simulink model "adaptive_backstepping_compliant_two_motor"  (R2022b)
settings: Solver=VariableStepAuto  StartTime=0.0  StopTime=80  RelTol=1e-3
values from neighbouring files (symbols this model uses):
  Lamda = 0.1*eye(2)    [init.m]
undefined symbols (not defined in the file or in its folder): D, J
settings Model: Creator=alexi  LastModifiedBy=alexi

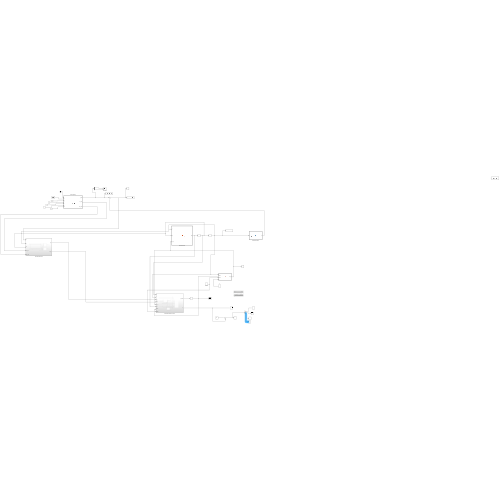
[thumbnail: Simulink's stored preview of the top-level diagram]
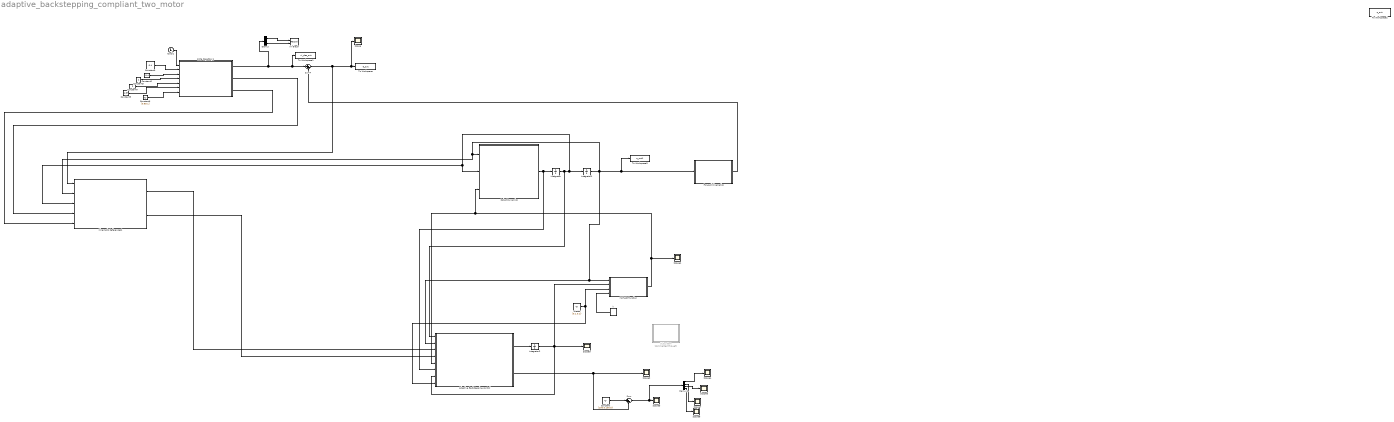
== system adaptive_backstepping_compliant_two_motor ==
  Adaptive Backstepping control : Subsystem
  Clock1 : Clock
  Constant : Constant  Value=[100,0,100,0]'
  Constant2 : Constant  Value=0.4
  Constant3 : Constant
  Constant4 : Constant  Value=2
  Constant5 : Constant  Value=1.57
  Constant6 : Constant  Value=[0.85,1]
  Constant9 : Constant  Value=0.4
  Demux : Demux  Outputs=2
  Demux1 : Demux
  Forward Kinematics : MATLAB Function  TreatAsAtomicUnit=on
  Integrator : Integrator  InitialCondition=[0,0]'
  Integrator1 : Integrator  InitialCondition=[0.1,0.1]'
  Integrator2 : Integrator  InitialCondition=[0.1,0.1]'
  Kinematic References1 : Subsystem
  MATLAB Function : MATLAB Function  TreatAsAtomicUnit=on
  Robot Dynamics : MATLAB Function  TreatAsAtomicUnit=on
  Scope{,1..8} (9 alike) : Scope
  Subsystem : Subsystem  Commented=through
  Sum : Sum  Inputs=|+-
  Sum4 : Sum  Inputs=|+-
  To Workspace : ToWorkspace  VariableName=e_out  SaveFormat=Timeseries  SampleTime=-1
  To Workspace1 : ToWorkspace  VariableName=xi_des_out  SaveFormat=Timeseries  SampleTime=-1
  To Workspace2 : ToWorkspace  VariableName=q_out  SaveFormat=Timeseries  SampleTime=-1
  To Workspace3 : ToWorkspace  VariableName=q_out1  SaveFormat=Timeseries  SampleTime=-1
  XY Graph : Record  FileSettingsInternal="{\"entries\":[{\"content\":{\"excelSettings\":{\"content\":{},\"type\":\"Streamout.ExcelSettings\"}},\"type\":\"Streamout.FileSettingStorage\",\"uuid\":\"f4627d21-b28b-402b-bd08-974ef3759845\"}],\"packageUris\":[\"http://schema.mathworks.com/mf0/streamout_blocks/R2020a\"],\"version\":\"1.0\"}"  Layout=[1 1]  SignalsInternal="{\"entries\":[{\"content\":{\"signals\":[{\"content\":{\"blockPath\":[\"adaptive_backstepping_compliant_two_motor/XY Graph\"],\"channel\":[],\"dimensions\":[1],\"domain\":\"adaptive_backstepping_compliant_two_motor/XY Graph\",\"lineColor\":\"#a2142f\",\"plots\":[1],\"port\":1,\"sid\":[\"\"],\"signalID\":23927,\"signalName\":\"Demux:1\"},\"type\":\"RecordBlkView.Signal\",\"uuid\":\"3e1d4046-1d32-4535-a7c4-decc746449ac\"},{\"content\":{\"blockPath\":[\"adaptive_backstepping_compliant_two_motor/XY Graph\"],\"channel\":[],\"dimensions\":[1],\"domain\":\"adaptive_backstepping_compliant_two_motor/XY Graph\",\"lineColor\":\"#139fff\",\"plots\":[1],\"port\":2,\"sid\":[\"\"],\"signalID\":23931,\"signalName\":\"Demux:2\"},\"type\":\"RecordBlkView.Signal\",\"uuid\":\"5c0d9346-56f9-4433-aa2f-4cb85fd46017\"}]},\"type\":\"RecordBlkView.InputSignals\",\"uuid\":\"d653fb0d-02e5-43c7-a84f-fb5375aaeae1\"}],\"packageUris\":[\"http://schema.mathworks.com/mf0/streamout_blocks/R2020a\"],\"version\":\"1.0\"}"  VisualizationBindings="{\"xyplotplugin\":{\"info\":[{\"series\":[{\"bindingParametersList\":[{\"parameter\":\"X-Axis\",\"signalID\":23927,\"signalName\":\"Demux:1\"},{\"parameter\":\"Y-Axis\",\"signalID\":23931,\"signalName\":\"Demux:2\"}],\"seriesID\":46846}],\"subplotID\":1}]}}"  CompatibilityTag=XY
  circle trajectory1 : MATLAB Function  TreatAsAtomicUnit=on
  k : Constant  Value=[100 0 50 0]'
  thetad : Constant  Value=[0.1,0.1]'
  wires:
  circle trajectory1/2(dxi_des) -> Kinematic References1/4(dxi_des)
  MATLAB Function/1(tau_el) -> Scope1/1, Robot Dynamics/3(tau_el), Adaptive Backstepping control/5(tau_el)
  circle trajectory1/3(ddxi_des) -> Kinematic References1/5(ddxi_des)
  thetad/1 -> Adaptive Backstepping control/8(thetad), MATLAB Function/3(thetad)
  circle trajectory1/1(xi_des) -> Demux/1, To Workspace1/1, Sum4/1
  Robot Dynamics/1(ddq) -> Adaptive Backstepping control/6(ddq), Integrator/1
  Demux/1 -> XY Graph/1
  Kinematic References1/2(ddq_r) -> Adaptive Backstepping control/4(ddq_r)
  Adaptive Backstepping control/1(d_thetas) -> Integrator2/1
  Kinematic References1/1(dq_r) -> Adaptive Backstepping control/3(dq_r)
  Integrator/1 -> Adaptive Backstepping control/1(dq), Integrator1/1, Robot Dynamics/2(dq), Kinematic References1/3(dq)  "dq"
  Forward Kinematics/1(xi) -> Sum4/2  "xi"
  Integrator2/1 -> Scope5/1, Adaptive Backstepping control/7(thetas), MATLAB Function/2(thetas)
  Sum4/1 -> Scope/1, To Workspace/1, Kinematic References1/1(e)
  Integrator1/1 -> Adaptive Backstepping control/2(q), MATLAB Function/1(q), Forward Kinematics/1(q), To Workspace3/1, Kinematic References1/2(q), Robot Dynamics/1(q)  "q"
  Adaptive Backstepping control/2(pi) -> Sum/2, Scope2/1
  Constant/1 -> Sum/1
  Sum/1 -> Demux1/1, Scope3/1
  Constant3/1 -> circle trajectory1/4(a)
  Constant4/1 -> circle trajectory1/5(b)
  Constant9/1 -> circle trajectory1/2(A)
  Constant2/1 -> circle trajectory1/3(B)
  Clock1/1 -> circle trajectory1/1(t)
  Constant6/1 -> circle trajectory1/7(p0)
  Constant5/1 -> circle trajectory1/6(d)
  Demux/2 -> XY Graph/2
  k/1 -> MATLAB Function/4(pi)
  Demux1/1 -> Scope4/1
  Demux1/3 -> Scope6/1
  Demux1/2 -> Scope7/1
  Demux1/4 -> Scope8/1

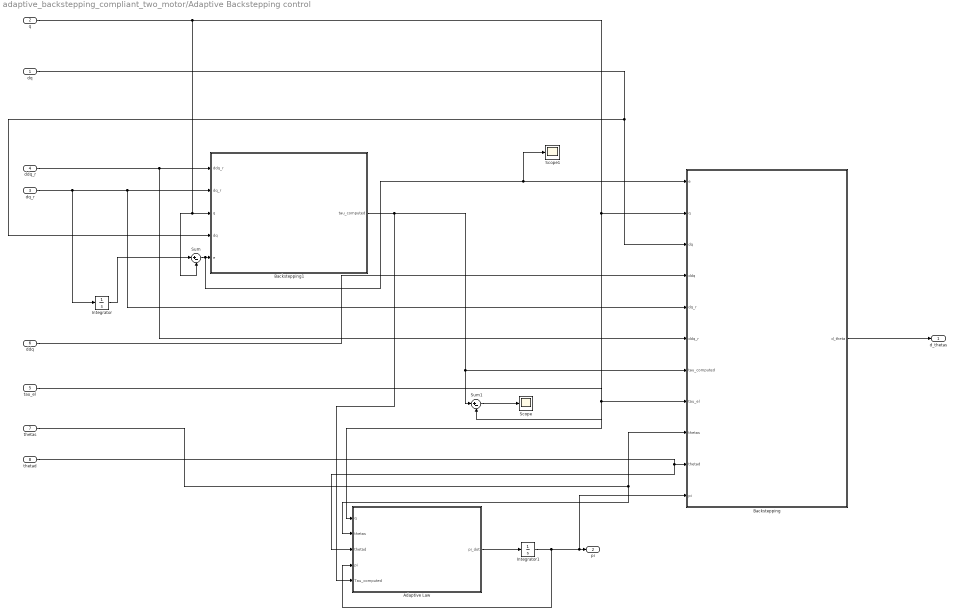
== system adaptive_backstepping_compliant_two_motor/Adaptive Backstepping control ==
  dq : Inport
  q : Inport  Port=2
  dq_r : Inport  Port=3
  ddq_r : Inport  Port=4
  tau_el : Inport  Port=5
  ddq : Inport  Port=6
  thetas : Inport  Port=7
  thetad : Inport  Port=8
  Adaptive Law : MATLAB Function  TreatAsAtomicUnit=on
  Backstepping : MATLAB Function  TreatAsAtomicUnit=on
  Backstepping1 : MATLAB Function  TreatAsAtomicUnit=on
  Integrator : Integrator  InitialCondition=[0.1,0.1]'
  Integrator1 : Integrator  InitialCondition=[130, -0.3, 51, -0.3]'
  Scope : Scope
  Scope1 : Scope
  Sum : Sum  Inputs=|+-
  Sum1 : Sum  Inputs=|+-
  d_thetas : Outport
  pi : Outport  Port=2
  wires:
  dq_r/1 -> Integrator/1, Backstepping1/2(dq_r), Backstepping/5(dq_r)
  q/1 -> Adaptive Law/1(q), Backstepping/2(q), Backstepping1/3(q), Sum/2
  Backstepping1/1(tau_computed) -> Adaptive Law/5(Tau_computed), Sum1/1, Backstepping/7(tau_computed)
  tau_el/1 -> Sum1/2, Backstepping/8(tau_el)
  ddq_r/1 -> Backstepping/6(ddq_r), Backstepping1/1(ddq_r)
  dq/1 -> Backstepping1/4(dq), Backstepping/3(dq)
  Backstepping/1(d_theta) -> d_thetas/1
  ddq/1 -> Backstepping/4(ddq)
  thetas/1 -> Adaptive Law/2(thetas), Backstepping/9(thetas)
  Integrator/1 -> Sum/1
  Sum/1 -> Scope1/1, Backstepping/1(e), Backstepping1/5(e)
  thetad/1 -> Adaptive Law/3(thetad), Backstepping/10(thetad)
  Sum1/1 -> Scope/1
  Adaptive Law/1(pi_dot) -> Integrator1/1
  Integrator1/1 -> Adaptive Law/4(pi), Backstepping/11(pi), pi/1

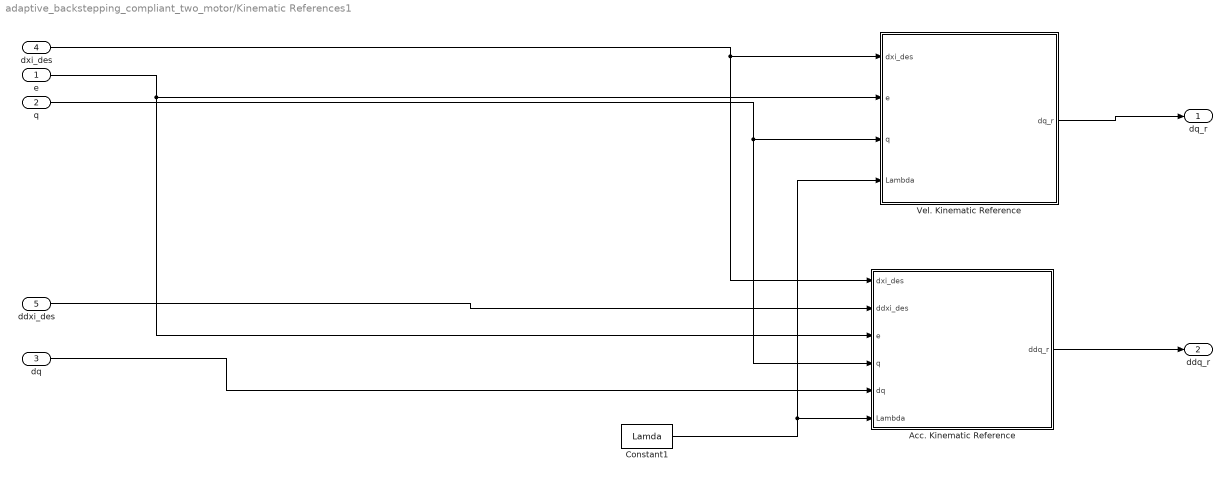
== system adaptive_backstepping_compliant_two_motor/Kinematic References1 ==
  e : Inport
  q : Inport  Port=2
  dq : Inport  Port=3
  dxi_des : Inport  Port=4
  ddxi_des : Inport  Port=5
  Acc. Kinematic Reference : MATLAB Function  TreatAsAtomicUnit=on
  Constant1 : Constant  Value=Lamda
  "Vel. Kinematic Reference " : MATLAB Function  TreatAsAtomicUnit=on
  dq_r : Outport  VectorParamsAs1DForOutWhenUnconnected=off
  ddq_r : Outport  Port=2  VectorParamsAs1DForOutWhenUnconnected=off
  wires:
  ddxi_des/1 -> Acc. Kinematic Reference/2(ddxi_des)
  e/1 -> Acc. Kinematic Reference/3(e), "Vel. Kinematic Reference "/2(e)
  dxi_des/1 -> Acc. Kinematic Reference/1(dxi_des), "Vel. Kinematic Reference "/1(dxi_des)
  Constant1/1 -> "Vel. Kinematic Reference "/4(Lambda), Acc. Kinematic Reference/6(Lambda)
  "Vel. Kinematic Reference "/1(dq_r) -> dq_r/1
  dq/1 -> Acc. Kinematic Reference/5(dq)
  q/1 -> Acc. Kinematic Reference/4(q), "Vel. Kinematic Reference "/3(q)
  Acc. Kinematic Reference/1(ddq_r) -> ddq_r/1

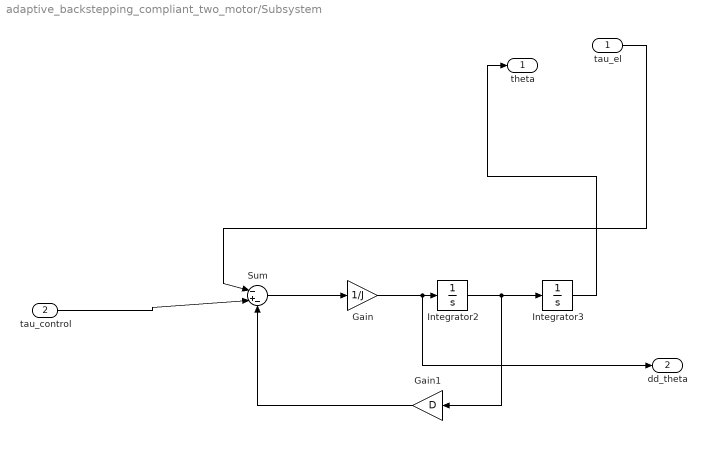
== system adaptive_backstepping_compliant_two_motor/Subsystem ==
  tau_el : Inport
  tau_control : Inport  Port=2
  Gain : Gain  Gain=1/J
  Gain1 : Gain  Gain=D
  Integrator2 : Integrator
  Integrator3 : Integrator
  Sum : Sum  Inputs=|-+-
  theta : Outport
  dd_theta : Outport  Port=2
  wires:
  tau_control/1 -> Sum/2
  Integrator3/1 -> theta/1
  Integrator2/1 -> Gain1/1, Integrator3/1
  Gain1/1 -> Sum/3
  Gain/1 -> dd_theta/1, Integrator2/1
  Sum/1 -> Gain/1
  tau_el/1 -> Sum/1

== matlab function adaptive_backstepping_compliant_two_motor/Adaptive Backstepping control/Adaptive Law ==
  data: q input; thetas input; thetad input; pi input; pi_dot output; Tau_computed input; R parameter
function pi_dot = fcn(q,thetas,thetad,pi,Tau_computed,R)
Kc = 300*eye(2);
Y = RR_Regression_Matrix_two_motors(q,thetas,thetad);
pi_dot = inv(R)*(Y'*Kc*Tau_computed-Y'*Kc*Y*pi);

== matlab function adaptive_backstepping_compliant_two_motor/Kinematic References1/Acc. Kinematic Reference ==
  data: dxi_des input; ddq_r output; ddxi_des input; e input; q input; dq input; Lambda input
function ddq_r = acc_kinematic_reference(dxi_des, ddxi_des, e, q, dq, Lambda)

coder.extrinsic('disp');

J = zeros(2,2);
dJ = zeros(2,2);

dq1 = dq(1);
dq2 = dq(2);

q1 = q(1);
q2 = q(2);

a1 = 1;
a2 = 1;

% Computing jacobian and derivative
J = [-a2*sin(q1 + q2) - a1*sin(q1), -a2*sin(q1 + q2);
      a2*cos(q1 + q2) + a1*cos(q1),  a2*cos(q1 + q2)];

dJ = [-a2*cos(q1 + q2)*(dq1 + dq2)-a1*cos(q1)*dq1, -a2*cos(q1 + q2)*(dq1 + dq2);
    -a2*sin(q1 + q2)*(dq1 + dq2)-a1*sin(q1)*dq1, -a2*sin(q1 + q2)*(dq1 + dq2)];

ddq_r = inv(J) * (ddxi_des + Lambda*dxi_des - Lambda*J*dq) ...
- inv(J)*dJ*inv(J)*(dxi_des + Lambda*e);
end

== matlab function adaptive_backstepping_compliant_two_motor/Kinematic References1/Vel. Kinematic Reference  ==
  data: dxi_des input; dq_r output; e input; q input; Lambda input
function dq_r = vel_kinematic_reference(dxi_des, e, q, Lambda)
a1 = 1;
a2 = 1;

q1 = q(1);
q2 = q(2);

% Computing jacobian
J = [-a2*sin(q1 + q2) - a1*sin(q1), -a2*sin(q1 + q2);
      a2*cos(q1 + q2) + a1*cos(q1),  a2*cos(q1 + q2)];

dq_r = inv(J) * (dxi_des + Lambda*e);
end

== matlab function adaptive_backstepping_compliant_two_motor/Adaptive Backstepping control/Backstepping1 ==
  data: ddq_r input; dq_r input; q input; dq input; e input; tau_computed output
function tau_computed  = computed_torque(ddq_r,dq_r,q,dq,e)

coder.extrinsic('disp');
rel_err = 0;

de = dq_r-dq;
Kp = 35;
Kv = 12;

% Get dynamic matrices
B = RR_mass_matrix(q);
C = RR_coriolis_matrix(q,dq);
G = RR_gravity_vector(q);

% Adding uncertainty
B = B.*(1 + rel_err);
C = C.*(1 + rel_err);
G = G.*(1 + rel_err);

% Control law
tau_computed = -(B*ddq_r+C*dq+G+B*Kp*e+B*Kv*de);

== matlab function adaptive_backstepping_compliant_two_motor/circle trajectory1 ==
  data: t input; xi_des output; dxi_des output; A input; B input; a input; b input; d input; p0 input; ddxi_des output
function [xi_des, dxi_des, ddxi_des] = lissajous(t,A,B,a,b,d,p0)

xi_des = [A*sin(a*t+d); B*sin(b*t)] + p0;
dxi_des = [A*a*cos(a*t+d); B*b*cos(b*t)];
ddxi_des = [-A*a^2*sin(a*t+d); -B*b^2*sin(b*t)];
% R = 0.2;
% xi_des = [R*(t - sin(2*t+pi)); R*(1-cos(2*t+pi))];
% dxi_des = [R - 2*R*cos(2*t+pi); 2*R*sin(2*t+pi)];
% ddxi_des = [4*R*sin(2*t+pi); 4*R*cos(2*t+pi)];

== matlab function adaptive_backstepping_compliant_two_motor/MATLAB Function ==
  data: q input; tau_el output; thetas input; thetad input; pi input
function tau_el = tau_elastica(q,thetas,thetad,pi)
% k = 0.1;
% a = 9;
k1_hat = pi(1);
k2_hat = pi(2);
k3_hat = pi(3);
k4_hat = pi(4);


tau_el1 = k1_hat*(q(1)-thetas(1)-thetad(1)) + k1_hat*(q(1) - thetas(1) + thetad(1)) + k2_hat*(q(1)-thetas(1) - thetad(1))^2 + k2_hat*(q(1)-thetas(1) + thetad(1))^2 + k3_hat*(q(1)-thetas(1) - thetad(1))^3 + k3_hat*(q(1)-thetas(1) + thetad(1))^3 + k4_hat*(q(1)-thetas(1) - thetad(1))^4 + k4_hat*(q(1)-thetas(1) + thetad(1))^4;
tau_el2 = k1_hat*(q(2)-thetas(2)-thetad(2)) + k1_hat*(q(2) - thetas(2) + thetad(2)) + k2_hat*(q(2)-thetas(2) - thetad(2))^2 + k2_hat*(q(2)-thetas(2) + thetad(2))^2 + k3_hat*(q(2)-thetas(2) - thetad(2))^3 + k3_hat*(q(2)-thetas(2) + thetad(2))^3 + k4_hat*(q(2)-thetas(2) - thetad(2))^4 + k4_hat*(q(2)-thetas(2) + thetad(2))^4;
tau_el = [tau_el1;tau_el2];

== matlab function adaptive_backstepping_compliant_two_motor/Adaptive Backstepping control/Backstepping ==
  data: e input; q input; dq input; ddq input; dq_r input; ddq_r input; tau_computed input; d_theta output; tau_el input; thetas input; thetad input; pi input
function d_theta  = backstepping(e,q,dq,ddq,dq_r,ddq_r,tau_computed,tau_el,thetas,thetad,pi)

coder.extrinsic('disp');
rel_err = 0;
de = dq_r-dq;
dde = ddq_r-ddq;
P = 5*eye(2);
K = 0.1;
Kc = 300;
Kp = 35;
Kv = 12;
a = 9;
k1_hat = pi(1);
k2_hat = pi(2);
k3_hat = pi(3);
k4_hat = pi(4);

% Get dynamic matrices
B = RR_mass_matrix(q);
C = RR_coriolis_matrix(q,dq);
G = RR_gravity_vector(q);

% Adding uncertainty
B = B.*(1 + rel_err);
C = C.*(1 + rel_err);
G = G.*(1 + rel_err);
g = [zeros(2,2); pinv(B)];
d_tau = C*dde-B*Kv*dde-B*Kp*de;

a1 = 1;
a2 = 1;



% Control law
%d_theta = B*ddq_r + C*dq_r + G + Ks*de + J.'*e;
Vx1 = [e'*Kp,de'];

l1 = -k1_hat - k1_hat - 2*k2_hat*(q(1)-thetas(1)-thetad(1)) - 2*k2_hat*(q(1)-thetas(1) + thetad(1)) - 3*k3_hat*(q(1)-thetas(1)-thetad(1))^2 - 3*k3_hat*(q(1)-thetas(1)+thetad(1))^2 - 4*k4_hat*(q(1)-thetas(1)-thetad(1))^3 - 4*k4_hat*(q(1)-thetas(1)+thetad(1))^3 ;
l2 = -k1_hat - k1_hat - 2*k2_hat*(q(2)-thetas(2)-thetad(2)) - 2*k2_hat*(q(2)-thetas(2) + thetad(2)) - 3*k3_hat*(q(2)-thetas(2)-thetad(2))^2 - 3*k3_hat*(q(2)-thetas(2)+thetad(2))^2 - 4*k4_hat*(q(2)-thetas(2)-thetad(2))^3 - 4*k4_hat*(q(2)-thetas(2)+thetad(2))^3;


l = [l1 0; 0 l2];


h1 = k1_hat*dq(1) + k1_hat*dq(1) + 2*k2_hat*(q(1)-thetas(1)-thetad(1))*dq(1) + 2*k2_hat*(q(1)-thetas(1)+thetad(1))*dq(1) + 3*k3_hat*dq(1)*(q(1)-thetas(1)-thetad(1))^2 + 3*k3_hat*dq(1)*(q(1)-thetas(1)+thetad(1))^2 + 4*k4_hat*dq(1)*(q(1)-thetas(1)-thetad(1))^3 + 4*k4_hat*dq(1)*(q(1)-thetas(1)+thetad(1))^3;
h2 = k1_hat*dq(2) + k1_hat*dq(2) + 2*k2_hat*(q(2)-thetas(2)-thetad(2))*dq(2) + 2*k2_hat*(q(2)-thetas(2)+thetad(2))*dq(2) + 3*k3_hat*dq(2)*(q(2)-thetas(2)-thetad(2))^2 + 3*k3_hat*dq(2)*(q(2)-thetas(2)+thetad(2))^2 + 4*k4_hat*dq(2)*(q(2)-thetas(2)-thetad(2))^3 + 4*k4_hat*dq(2)*(q(2)-thetas(2)+thetad(2))^3;

h = [h1;h2];

v = d_tau+pinv(P)*(Kc*(tau_computed-tau_el)-g'*Vx1');
d_theta = inv(l)*(v-h);

== matlab function adaptive_backstepping_compliant_two_motor/Robot Dynamics ==
  data: q input; dq input; tau_el input; ddq output
function ddq = inverse_dynamics(q,dq, tau_el)

% Get dynamic matrices
B = RR_mass_matrix(q);
C = RR_coriolis_matrix(q,dq);
G = RR_gravity_vector(q);
ddq = pinv(B)*(-tau_el - C*dq - G);

== matlab function adaptive_backstepping_compliant_two_motor/Forward Kinematics ==
  data: q input; xi output
function xi  = RR_forward_kinematics(q)

    q1 = q(1);
    q2 = q(2);

    a1 = 1;
    a2 = 1;

    p0 = [0;0];
    p1 = [a1*cos(q1); a1*sin(q1)];
    xi = p1+[a2*cos(q1+q2);a2*sin(q1+q2)];
end
